simulink model "MCLV2_dsPIC33EP256MC506_externalOpAmp_DataLog_R2017a"  (Simulink 8.9)
settings: Solver=FixedStepDiscrete  StartTime=0.0  StopTime=inf  FixedStep=.00005  RelTol=1e-3  EnableMultiTasking=on
undefined symbols (not defined in the file): A4, A8, B5, B6, C10, C5, C6, D5, DiscIntNeverNeededParam, F0, F1, Max, ms, P20, P24, P53, P54, P97, Pin, PWMmax, Resol, us
libraries: MCHP_Blockset x19, simulink x16, simulink_need_slupdate x1
(part 1 of 2)
Description:
  | MCLV V2 board connected to DC motor through PWM [1 2]
  | PIM 33EP256MC506 with internal Op-Amp (populated with resistances)
  | 
  | LED D2 blink at 5Hz. LED D1 is the CPU busy flag
settings Model: SuppressorTable="22 serialization::archive 15 0 6 0 0 3 8 0 0 0 0 6 0 0 1 0 94 MCLV2_dsPIC33EP256MC506_externalOpAmp_DataLog_R2017a/Steps Large1/Counter Limited 0-1 @ 1.25Hz 0 6 0 0 2 8 0 0 0 0 6 40 SimulinkFixedPoint:util:Overflowoccurred 0 0 0 6 0  0  0 0 0 0 8 20160608 0 0 0 15 23 17 0 1 41 Simulink:DataType:WarningOverFlowDetected 0 0 0  0  8 20160608 0 15 23 17 0 1 1 0 73 MCLV2_dsPIC33EP256MC506_externalOpAmp_DataLog_R2017a/Counter Free-Running 2 8 0 40 SimulinkFixedPoint:util:Overflowoccurred 0 0 0  0  8 20160523 0 10 57 55 0 1 41 Simulink:DataType:WarningOverFlowDetected 0 0 0  0  8 20160523 0 10 57 55 0 1 1 0 93 MCLV2_dsPIC33EP256MC506_externalOpAmp_DataLog_R2017a/Steps Large/Counter Limited 0-1 @ 1.25Hz 2 8 0 40 SimulinkFixedPoint:util:Overflowoccurred 0 0 0  0  8 20160608 0 15 23 17 0 1 41 Simulink:DataType:WarningOverFlowDetected 0 0 0  0  8 20160608 0 15 23 17 0 1"  Creator=R.Delpoux & L.Kerhuel  LastModifiedBy=Lubin Kerhuel
settings DataIOCC: LimitDataPoints=off  SaveFormat=Dataset  SignalLoggingSaveFormat=Dataset
settings OptimizationCC: DefaultParameterBehavior=Inlined  DefaultUnderspecifiedDataType=single  BooleansAsBitfields=on  PassReuseOutputArgsAs=Individual arguments  LifeSpan=auto
settings DebuggingCC: UnderspecifiedInitializationDetection=Simplified  MergeDetectMultiDrivingBlocksExec=error  MultiTaskCondExecSysMsg=none  ParameterOverflowMsg=warning  ParameterTunabilityLossMsg=error  FcnCallInpInsideContextMsg=error  StateNameClashWarn=none  SFUnexpectedBacktrackingDiag=error  SFNoUnconditionalDefaultTransitionDiag=error  SFExecutionAtInitializationDiag=warning
settings HardwareCC: ProdBitPerInt=16  ProdBitPerPointer=16  ProdBitPerSizeT=16  ProdBitPerPtrDiffT=16  ProdLargestAtomicInteger=Integer  ProdIntDivRoundTo=Zero  ProdEndianess=LittleEndian  ProdWordSize=16  ProdHWDeviceType=Generic->Custom
settings ModelReferenceCC: ModelReferenceNumInstancesAllowed=Single  PropagateSignalLabelsOutOfModel=on
settings SFSimCC: MATLABDynamicMemAlloc=off
settings RTWCC: SystemTargetFile=MCHP_dsPIC_stf.tlc  TemplateMakefile=MCHP_dsPIC.tmf  Description=Microchip Embedded Target PIC24 dsPIC30 dsPIC33 (real-time)  GenerateReport=on  IncludeHyperlinkInReport=on  LaunchReport=on  GenerateTraceInfo=on  GenerateTraceReport=on  GenerateTraceReportSl=on  GenerateTraceReportSf=on  GenerateTraceReportEml=on  GenerateCodeReplacementReport=on
settings CodeAppCC: ForceParamTrailComments=on  IgnoreCustomStorageClasses=off  MaxIdLength=255  OperatorAnnotations=on  SimulinkDataObjDesc=on  SFDataObjDesc=on  MATLABFcnDesc=on  InsertBlockDesc=on  MATLABSourceComments=on
settings STFCustomTargetCC: TargetLibSuffix=_lib.a  CodeReplacementLibrary=Microchip Code Replacement Library for dsPIC  MultiwordLength=256  IncludeMdlTerminateFcn=off  CombineOutputUpdateFcns=on  CombineSignalStateStructs=on  SuppressErrorStatus=on  ERTCustomFileBanners=on  SupportContinuousTime=off  RemoveResetFunc=on  MATLABClassNameForMDSCustomization=Simulink.SoftwareTarget.ERTCustomization  GRTInterface=off  SystemTargetFile=MCHP_dsPIC_stf.tlc
settings ERTTargetCC: TargetLibSuffix=_lib.a  CodeReplacementLibrary=Microchip Code Replacement Library for dsPIC  ParMdlRefBuildCompliant=off  CompOptLevelCompliant=off  ConcurrentExecutionCompliant=off  IncludeMdlTerminateFcn=off  CombineSignalStateStructs=on  SuppressErrorStatus=on  SupportNonInlinedSFcns=on  ModelStepFunctionPrototypeControlCompliant=off  CPPClassGenCompliant=off  UseToolchainInfoCompliant=off  ExtModeStaticAllocSize=500  InlinedParameterPlacement=NonHierarchical  ERTSrcFileBannerTemplate=MCHP_dsPIC_code_template.cgt  ERTHdrFileBannerTemplate=MCHP_dsPIC_code_template.cgt  ERTDataSrcFileTemplate=MCHP_dsPIC_code_template.cgt  ERTDataHdrFileTemplate=MCHP_dsPIC_code_template.cgt  ERTCustomFileTemplate=MCHP_main.tlc
settings CustomProperty: DataType=string  Value=33EP256MC506
settings EnumStrPairs: String=elf
settings ConfigComp: CovMetricSettings=dwe  CovHtmlReporting=off  CovSaveCumulativeToWorkspaceVar=off  CovSaveSingleToWorkspaceVar=off  CovExternalEMLEnable=on

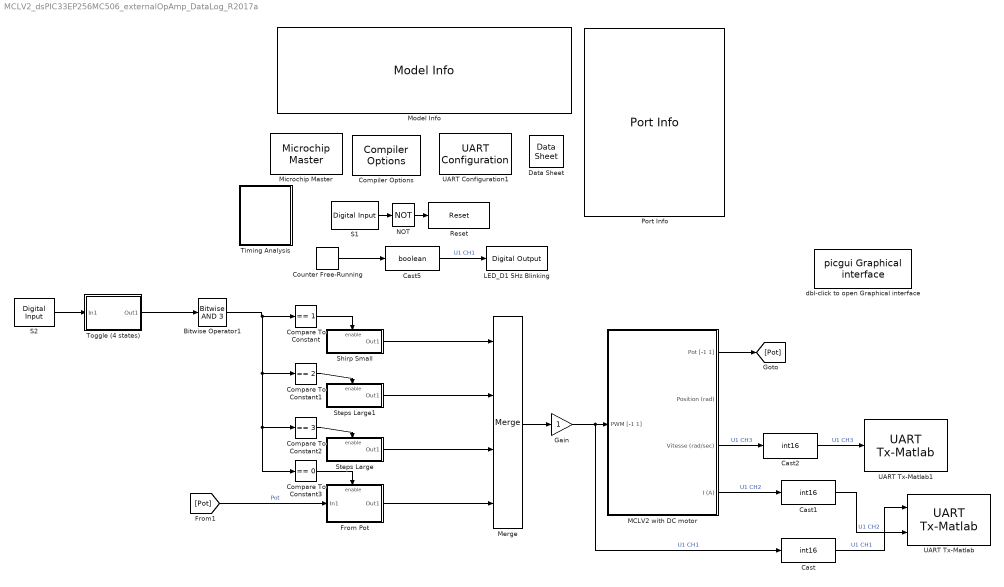
== system MCLV2_dsPIC33EP256MC506_externalOpAmp_DataLog_R2017a ==
  Bitwise Operator1 : simulink/Logic and Bit Operations/Bitwise Operator  logicop=AND  UseBitMask=on  BitMask=3  BitMaskRealWorld=Stored Integer
  Cast : DataTypeConversion  OutDataTypeStr=int16  ConvertRealWorld=Stored Integer (SI)
  Cast1 : DataTypeConversion  OutDataTypeStr=int16  ConvertRealWorld=Stored Integer (SI)
  Cast2 : DataTypeConversion  OutDataTypeStr=int16  ConvertRealWorld=Stored Integer (SI)
  Cast5 : DataTypeConversion  OutDataTypeStr=boolean
  Compare To Constant : simulink/Logic and Bit Operations/Compare To Constant  relop===  const=1  OutDataTypeStr=boolean
  Compare To Constant1 : simulink/Logic and Bit Operations/Compare To Constant  relop===  const=2  OutDataTypeStr=boolean
  Compare To Constant2 : simulink/Logic and Bit Operations/Compare To Constant  relop===  const=3  OutDataTypeStr=boolean
  Compare To Constant3 : simulink/Logic and Bit Operations/Compare To Constant  relop===  const=0  OutDataTypeStr=boolean
  Compiler Options : MCHP_Blockset/System Configuration/Compiler Options  Priority=1  LATEST_CMPLR=on  COMP_LIST=Dynamic Options  COMP_LIST_TXT=xc16 - v1.35  USE_64BIT_DOUBLE=off  MCHP_MULTITHREAD_COMPILATION=on  UseCustom_LinkerScript=off  MCHP_MASTERLINK=MCLV2_dsPIC33EP256MC506_externalOpAmp_DataLog_R2017a/Microchip Master  OPTIMIZATION_LEVEL=1  MPLAB_LINKLIB=default  MPLAB_LINKLIB1=default  UNROLL_LOOPS=on  OMIT_FRAME_POINTER=off  PROCEDURAL_ABSTRACTION=off  MCONST=in code memory  MDATA=Use only memory below address 8192 (faster)  MSCALAR=Use only memory below address 8192 (faster)  MCODE=is less than 32768 (faster)  HEAP_SIZE=0  OMF=elf  DEBUG_INFO=on  AssemblyListing=on  ProduceHexOutput=off
      settings: SourceProductName=MPLAB Device Blocks for Simulink
  Counter Free-Running : simulink/Sources/Counter Free-Running  NumBits=1  tsamp=.1
  Data Sheet : MCHP_Blockset/System Info/Data Sheet  DOC_Type=datasheet  DOC_MCHP_Id=33FJ64MC802  DOC_FileLastCheckTime=[0 0 0 0 0 0]  cpy_MCHP_Id=33EP256MC506  MCHP_MASTERLINK=MCLV2_dsPIC33EP256MC506_externalOpAmp_DataLog_R2017a/Microchip Master
      settings: AttributesFormatString=%<cpy_MCHP_Id>  SourceProductName=MPLAB Device Blocks for Simulink
  From Pot : Subsystem
  Gain : Gain  SaturateOnIntegerOverflow=on  OutDataTypeStr=Inherit: Same as input
  LED_D1 5Hz Blinking : MCHP_Blockset/Digital IO/Digital Output  PORT=Dynamic Options  PORT_TXT="D   [ 5  6  8 ]"  PIN=6  PACK=off  SIMULTANEOUS=off  READPREVIOUS=off  ORDERING=None  SampleTime=-1  MCHP_MASTERLINK=MCLV2_dsPIC33EP256MC506_externalOpAmp_DataLog_R2017a/Microchip Master
      settings: SourceProductName=MPLAB Device Blocks for Simulink
  MCLV2 with DC motor : Subsystem
  Merge : Merge  Inputs=4
  Microchip Master : MCHP_Blockset/System Configuration/Microchip Master  Priority=1  PICREF=33EP256MC506  TIMESTEP_REF=ADC  BUSYFLAG=Dynamic Options  BUSYFLAG_TXT=None  PWRTEN=Not used  BOREN=Disable  BODENV=2.7V  BORV=Not used  FPWRT=128ms  DSBOREN=Enable ZPBOR during Deep Sleep Mode  DSLPBOR=Not used  MCLRE=Enabled  SMCLR=MCLR pin generates a normal system Reset  PMDL1WAY=Allow only one reconfiguration  RSTPRI=Device will obtain reset instruction from Primary flash  TEMP=Not used  SOSCSRC=Not used  SOSCSEL=Not used  IOL1WAY=Allow only one reconfiguration  ALTVREF=Not used  DISUVREG=Not used  DSSWEN=Not used  LPCFG=Not used  RTCBAT=Not used  VBTBOR=Not used  WUTSEL=Not used  POWERSAVE=off  FNOSC=Primary Oscillator (XT; HS; EC)  FPR=ECIO w/ PLL 16x  FOSFPR=HS3 w/PLL 16x  FOS=Primary Oscillator  FRANGE=High Range  OSCILLATOR_SELECT=Crystal / Ceramic resonator  OSCILLATOR_SELECT_spd=Crystal / Ceramic resonator  QUARTZ=8e6  QUARTZ_spd=8e6  POSCGAIN=2x gain setting  POSCBOOST=Boost the kick start of the oscillator  SOSCGAIN=2x gain setting  SOSCBOOST=Boost the kick start of the oscillator  ACTIV_PLL=on  ACTIV_PLL_spd=on  MIPS_DESIRED=70e6  MIPS_DESIRED_spd=70e6  FPLLMUL=Not used  FPLLIDIV=8x Divider  POSCFREQ=Not used  POSCMD=XT Crystal Oscillator Mode  POSCMOD=Primary osc disabled  MIPS=70 * 1e6  ACLKCON=Optimized for PWM resolution & ADC conversion speed  FPLLODIV=32x Divider  PLLKEN=Clock switch to PLL source will wait until the PLL lock signal is valid.  FCKSM=Clock switching is enabled;Fail-safe Clock Monitor is disabled  FCKSMEN=Sw Disabled; Mon Disabled  IESO=Start up with FRC; then switch  DSWDTPS=1:2^36  FWDTEN=Disable  FWDTWINSZ=Window size is 25%  FWPSA=1:512  FWPSA0=1:128  FWPSB=1:16  WDT=Disable  WDTPOST=1:32768  WDTPRE=1:128  WDTPS=1:1048576  WINDIS=Watchdog Timer in Non-Window mode  WWDTEN=Non-Window mode  DSWDTEN=Enable DSWDT during Deep Sleep Mode  DSWDTOSC=Select LPRC as DSWDT Reference clock  FPBDIV=Not used  FSOSCEN=Enable SOSC  LPRCSEL=Not used  OSCIOFCN=Not used  OSCIOFNC=general purpose digital I/O pin  LVRCFG=Not used  PLL_96MHZ=Not used  PLL96MHZ=Not used  PLLDIV=Not used  WDTCLK=Not used  WDTCMX=Not used  WDTWIN=WDT Window is 25% of WDT period  APL=Aux Flash Code protect is disabled  APLK=Aux Flash Write Protection or Code Protection is Enabled  AWRP=Auxiliary program memory is not write-protected  BSS=No Boot program Flash segment  BWP=Not used  BWRP=Boot Segment may be written  CP=Protection Disabled  EBS=No Boot EEPROM  ESS=No Segment Data EEPROM  GCP=General Segment Code protect is Disabled  GSS=General Segment Code protect is Disabled  GSS0=Not used  GSSK=General Segment Write Protection or Code Protection is Enabled  GWRP=General Segment may be written  PWP=Not used  RBS=No Boot RAM  RSS=No Secure RAM  SSS=No Secure Segment  SWRP=Secure segment may be written  WPCFG=Not used  WPDIS=Not used  WPEND=Not used  WPFP=Not used  ICESEL=Communicate on PGEC1/PGED1  ICS=Communicate on PGEC2 and PGED2  JTAGEN=Disable  COE=Not used  RES=Not used  DEBUG=Debugger is disabled  BACKBUG=Not used  BKBUG=Not used  ALTI2C=I2C mapped to SDA1/SCL1 pins  ALTI2C1=I2C1 mapped to SDA1/SCL1 pins  ALTI2C2=I2C2 mapped to SDA2/SCL2 pins  ALTQIO=QEA1; QEB1; INDX1 are selected as inputs to QEI1  ALTSS1=SS1A is selected as the I/O pin for SPI1  CMPPOL0=Hysteresis is applied to falling edge  CMPPOL1=Hysteresis is applied to falling edge  FCANIO=Not used  FETHIO=Default Ethernet I/O  FMIIEN=MII Enabled  FSRSSEL=Not used  FUSBIDIO=Controlled by the USB Module  FVBUSONIO=Not used  HPOL=PWM module high side output pins have active-high output polarity  HYST0=45 mV Hysteresis  HYST1=45 mV Hysteresis  I2C1SEL=Not used  LPOL=PWM module low side output pins have active-high output polarity  PWMPIN=PWM module pins controlled by PORT register at device Reset  RTCOSC=Not used  UPLLEN=USB PLL Disabled  UPLLIDIV=Not used  ATMOD8=Not used  ALTPMP=Not used  I2C2SEL=Not used  ALTADREF=Not used  ALTCVREF=Not used  PWMLOCK=PWM registers may be written without key sequence  MCHP_TIMER_RESULT=[ ]  MCHP_PLLRegisters="[5    243  16385     -1]"  MCHPVAR=MCHP.fcy.MIPS=70000000;MCHP.fcy.SYSCLK=70000000;MCHP.fcy.ADC=70000000;MCHP.fcy.Comparator=70000000;MCHP.fcy.I2C=70000000;MCHP.fcy.SPI=70000000;MCHP.fcy.UART=70000000;MCHP.fcy.Timers=70000000;MCHP.fcy.OC=70000000;MCHP.fcy.IC=70000000;MCHP.fcy.Ports=70000000;MCHP.fcy.QEI=70000000;MCHP.PowerSave=0;MCHP.TimeStepFactor=-20000;MCHP.TimeStep_Timer=-1;MCHP.NTIMERS=5;MCHP.id.name='33EP256MC506';MCHP.id.N=reshape([33 256 506],1,3);MCHP.id.L=reshape({ 'EP','MC',''},1,3);MCHP.id.Arch=3;MCHP.periph.PPS.reg_RPINRx=reshape([-1 1 1 -1 -1 -1 1 -1 -1 -1 -1 -1 -1 -1 1 1 1 1 -1 -1 -1 -1 -1 -1 1 1 -1 -1 1 1 1 1 -1 -1 -1 -1 1 -1 1 -1 -1 -1 -1 -1 1 1 1 -1 -1 -1 -1 -1 1 -1 -1 -1 -1 -1 -1 -1 -1 -1 -1 -1 -1 -1 -1 -1 -1 -1 -1 -1 -1 -1 -1 1 -1 1 1 1],1,80);MCHP.PPS.dsPIC.RP=reshape([-1 -1 -1 -1 -1 -1 -1 -1 -1 -1 -1 -1 -1 -1 -1 -1 -1 -1 -1 -1 4 -1 -1 -1 -1 -1 -1 -1 -1 -1 -1 -1 -1 -1 -1 19 20 21 22 23 24 25 26 27 -1 -1 -1 -1 -1 -1 -1 -1 -1 -1 38 39 40 41 -1 -1 -1 -1 -1 -1 -1 -1 -1 -1 -1 -1 -1 -1 -1 -1 -1 -1 -1 -1 -1 -1 -1 -1 -1 -1 -1 -1 -1 -1 -1 -1 -1 -1 -1 -1 -1 -1 -1 81 -1 -1 -1 -1 -1 -1 -1 -1 -1 -1 -1 -1 -1 -1 -1 -1 -1 -1 -1 -1 102 -1 104],1,121);MCHP.PPS.dsPIC.RPI=reshape([-1 -1 -1 -1 -1 -1 -1 -1 -1 -1 -1 -1 -1 -1 -1 -1 -1 -1 -1 -1 -1 -1 -1 -1 8 9 -1 11 12 -1 -1 -1 16 17 18 -1 -1 -1 -1 -1 -1 -1 -1 -1 28 29 30 31 -1 -1 -1 35 36 37 -1 -1 -1 -1 42 -1 -1 -1 -1 -1 -1 -1 -1 -1 -1 -1 -1 -1 -1 -1 -1 -1 -1 -1 -1 -1 -1 -1 -1 -1 -1 -1 -1 -1 -1 -1 -1 -1 -1 -1 78 79 80 -1 -1 -1 -1 -1 -1 -1 -1 -1 -1 -1 -1 -1 -1 -1 -1 -1 -1 -1 -1 -1 -1 103 -1 105],1,122);MCHP.PPS.dsPIC.RPINR_list=reshape({ '1','INT1','INT2','INT3','INT4','T1CK','T2CK','T3CK','T4CK','T5CK','T6CK','T7CK','T8CK','T9CK','IC1','IC2','IC3','IC4','IC5','IC6','IC7','IC8','OCFA','OCFB','FLT1','FLT2','FLT3','FLT4','QEA1','QEB1','INDX1','HOME1','QEA2','QEB2','INDX2','HOME2','U1RX','U1CTS','U2RX','U2CTS','SDI1','SCK1_in','SS1_in','44','SDI2','SCK2_in','SS2_in','48','CSDIR','CSCK','COFS','52','C1RX','C2RX','U3RX','U3CTS','U4RX','U4CTS','SDI3','SCK3_in','SS3_in','62','SDI4','SCK4_in','SS4_in','66','IC9','IC10','IC11','IC12','IC13','IC14','IC15','IC16','OCFC','SYNCI1','SYNCI2','DTCMP1','DTCMP2','DTCMP3','DTCMP4','DTCMP5','DTCMP6','DTCMP7','FLT5','FLT6','FLT7','FLT8','89','SENT1','SENT2','92'},1,92);MCHP.PPS.dsPIC.RPOR_list=reshape({ '1','U1TX','U1RTS','U2TX','U2RTS','SDO1','SCK1_out','SS1_out','SDO2','SCK2_out','SS2_out','CSDO','CSCK','COFS','C1TX','C2TX','OC1','OC2','OC3','OC4','OC5','OC6','OC7','OC8','C1OUT','C2OUT','C3OUT','U3TX','U3RTS','U4TX','U4RTS','SDO3','SCK3_out','SS3_out','SDO4','SCK4_out','SS4_out','OC9','OC10','OC11','OC12','OC13','OC14','OC15','OC16','SYNCO1','SYNCO2','QEI1CCMP','QEI2CCMP','REFCLK','C4OUT','C5OUT','52','53','54','55','56','SENT1','SENT2'},1,59);MCHP.PPS.map_RPnR_RPORx=reshape([20 35 36 37 38 39 40 41 42 43 54 55 56 57 -1 97 -1 118 120],1,19);MCHP.Rx=reshape([13 15 21 -1 -1 58 -1 -1 -1 -1 -1 14 16 22 -1 -1 59 -1 -1 -1 -1 -1 -1 17 23 -1 -1 -1 -1 -1 -1 -1 -1 -1 18 35 -1 -1 -1 -1 -1 -1 -1 -1 33 32 36 -1 -1 -1 -1 -1 -1 -1 -1 -1 43 37 53 -1 -1 -1 -1 -1 -1 -1 -1 44 50 54 -1 -1 4 -1 -1 -1 -1 1 46 51 -1 -1 -1 5 -1 -1 -1 -1 31 48 52 42 -1 -1 6 -1 -1 -1 -1 34 49 55 -1 -1 -1 8 -1 -1 -1 -1 64 60 45 -1 -1 -1 -1 -1 -1 -1 -1 12 61 24 -1 -1 -1 -1 -1 -1 -1 -1 11 62 39 -1 27 -1 -1 -1 -1 -1 -1 -1 63 47 -1 28 -1 -1 -1 -1 -1 -1 -1 2 -1 -1 29 -1 -1 -1 -1 -1 -1 -1 3 40 -1 30 -1 -1 -1 -1 -1 -1],11,16);MCHP.ADC.ANtype=reshape([3 0],1,2);MCHP.ADC.ADCONx=reshape([47103 59391 40959 263 0 0],1,6);MCHP.ADC.ADCHS_0=reshape([40863 1799],1,2);MCHP.ADC.Flags=reshape([1 0],1,2);MCHP.ADC.Buffer=reshape([16 -1],1,2);MCHP.ADC.port=reshape([0 1 16 17 18 19 32 33 34 11 12 43 76 77 78 79 -1 -1 -1 -1 -1 -1 -1 -1 -1 -1 -1 -1 -1 -1 -1 -1 -1 -1 -1 -1 -1 -1 -1 -1 -1 -1 -1 -1 -1 -1 -1 -1 -1 -1 -1 -1 -1 -1 -1 -1 -1],1,57);MCHP.ADC.port_ALT=reshape([-1 -1 -1 -1],1,4);MCHP.ADC.port_VrefP=17;MCHP.ADC.port_VrefM=16;MCHP.ADC.port_AVdd=-1;MCHP.ADC.port_AVss=-1;MCHP.ADC.ADCDATA=reshape([0 0 0 0 0 0 0 0 0 0 0 0 0 0 0 0 0 0 0 0 0 0 0 0 0 0 0 0 0 0 0 0 0 0 0 0 0 0 0 0 0 0 0 0 0 0 0 0 0 0 0 0 0 0 0 0 0],1,57);MCHP.memory.RAM=32768;MCHP.memory.RAM_XBegin=4096;MCHP.memory.RAM_YBegin=20480;MCHP.memory.RAM_dma=reshape([-1 -1],1,2);MCHP.memory.FLASH_ECC=0;MCHP.DMA.Num=4;MCHP.DMA.CNTmax=16383;MCHP.QEI.QEICONx=reshape([49023 -1 -1 -1 -1 -1],1,6);MCHP.QEI.QEItype=1;MCHP.QEI.Port_QEI_INDX=reshape([-1 -1],1,2);MCHP.QEI.Port_QEI_QEA=reshape([-1 -1],1,2);MCHP.QEI.Port_QEI_QEB=reshape([-1 -1],1,2);MCHP.QEI.Port_QEI_UPDN=reshape([-1 -1],1,2);MCHP.INT.Port=reshape([23 32767 32767 -1 -1],1,5);MCHP.PWM_HS.Flags=reshape([3 1 0],1,3);MCHP.PWM.port_FLT=reshape([-1 -1 -1 34 43 -1 -1 -1 -1 -1 -1 -1 -1 -1 -1 -1 -1 -1 -1 -1 -1 -1 -1 -1 -1 -1 -1 -1 -1 -1 -1 -1 20],1,33);MCHP.PWM.PWMRef=-1;MCHP.PWM.Flag=0;MCHP.PWM.Port_PWM_l=reshape([31 -1 29 -1 27 -1 -1 -1 -1 -1 -1 -1 -1 -1 -1 -1 -1 -1 -1 -1 -1 -1 -1 -1],2,12);MCHP.PWM.Port_PWM_h=reshape([30 -1 28 -1 26 -1 -1 -1 -1 -1 -1 -1 -1 -1 -1 -1 -1 -1 -1 -1 -1 -1 -1 -1],2,12);MCHP.IC.Port=reshape([32767 32767 32767 32767 0 0 0 0 0 0 0 0 0 0 0 0],1,16);MCHP.IC.type=1;MCHP.OC.Port=reshape([32767 32767 32767 32767 0 0 0 0 0 0 0 0 0 0 0 0],1,16);MCHP.OC.type=1;MCHP.CN.Port=reshape([-1 -1 -1 -1 -1 -1 -1 -1 -1 -1 -1 -1 -1 -1 -1 -1 -1 -1 -1 -1 -1 -1 -1 -1 -1 -1 -1 -1 -1 -1 -1 -1 -1 -1 -1 -1 -1 -1 -1 -1 -1 -1 -1 -1 -1 -1 -1 -1 -1 -1 -1 -1 -1 -1 -1 -1 -1 -1 -1 -1 -1 -1 -1 -1 -1 -1 -1 -1 -1 -1 -1 -1 -1 -1 -1 -1 -1 -1 -1 -1 -1 -1 -1 -1 -1],1,85);MCHP.CN.PullUp=reshape([8083 65535 49151 352 61440 3 960 0 0 0 0],1,11);MCHP.CN.type=1;MCHP.CN.Flag_PullDown=1;MCHP.SPI.Refs=reshape([1 2 0 0 0 0],1,6);MCHP.SPI.SPIxCON1=8191;MCHP.SPI.SPIxCON2=57347;MCHP.SPI.Port_SDI=reshape([9 -1 -1 -1 -1 -1],1,6);MCHP.SPI.Port_SDO=reshape([4 -1 -1 -1 -1 -1],1,6);MCHP.SPI.Port_SCK=reshape([35 -1 -1 -1 -1 -1],1,6);MCHP.SPI.Port_SS=reshape([16 -1 -1 -1 -1 -1],1,6);MCHP.I2C.Refs=reshape([1 2 0 0 0],1,5);MCHP.I2C.I2CxCON=49151;MCHP.I2C.NewRegName=1;MCHP.I2C.Port_SDA=reshape([36 8 -1 -1 -1],1,5);MCHP.I2C.Port_SCL=reshape([37 20 -1 -1 -1],1,5);MCHP.I2C.Port_ASDA=reshape([25 21 -1 -1 -1],1,5);MCHP.I2C.Port_ASCL=reshape([24 22 -1 -1 -1],1,5);MCHP.I2C.Fuse_Port_SCL_SDA=reshape([3 1 4 1 -1 -1 -1 -1 -1 -1],2,5);MCHP.I2C.Fuse_Port_ASCL_ASDA=reshape([3 2 4 2 -1 -1 -1 -1 -1 -1],2,5);MCHP.PGA.Port_PGA1P=reshape([-1 -1 -1 -1],1,4);MCHP.PGA.Port_PGA1N=reshape([-1 -1 -1 -1],1,4);MCHP.PGA.Port_PGA2P=reshape([-1 -1 -1 -1],1,4);MCHP.PGA.Port_PGA2N=reshape([-1 -1 -1 -1],1,4);MCHP.PGA.Num=0;MCHP.HS_AnalogComparator.Port_CMP1=reshape([-1 -1 -1 -1],1,4);MCHP.HS_AnalogComparator.Port_CMP2=reshape([-1 -1 -1 -1],1,4);MCHP.HS_AnalogComparator.Port_CMP3=reshape([-1 -1 -1 -1],1,4);MCHP.HS_AnalogComparator.Port_CMP4=reshape([-1 -1 -1 -1],1,4);MCHP.HS_AnalogComparator.PORT_EXTREFx=reshape([-1 -1],1,2);MCHP.HS_AnalogComparator.Port_DACOUTx=reshape([-1 -1],1,2);MCHP.HS_AnalogComparator.Num=0;MCHP.Comp.Port_CVrefin=-1;MCHP.Comp.Port_CVref=-1;MCHP.Comp.Port_CVref1O=24;MCHP.Comp.Port_CVref2O=4;MCHP.Comp.Port_CxOUT=reshape([32767 32767 32767 32767 -1],1,5);MCHP.Comp.Port_OAxOUT=reshape([17 0 32 -1 -1],1,5);MCHP.Comp.Port_CxINP=reshape([18 1 34 32 -1],1,5);MCHP.Comp.Port_CxINM=reshape([19 43 -1 -1 16 76 -1 -1 33 77 -1 -1 33 -1 -1 -1 -1 -1 -1 -1],4,5);MCHP.Comp.nComp=reshape([4 0 0],1,3);MCHP.Comp.OpAmp=7;MCHP.Comp.CVRCON=reshape([17663 0],1,2);MCHP.CDAC.Port_DACx=reshape([-1 -1 -1],1,3);MCHP.CDAC.nCDAC=0;MCHP.UART.port_Rx=reshape([32767 32767 -1 -1 -1 -1],1,6);MCHP.UART.port_Tx=reshape([32767 32767 -1 -1 -1 -1],1,6);MCHP.UART.port_ARx=reshape([-1 -1],1,2);MCHP.UART.port_ATx=reshape([-1 -1],1,2);MCHP.UART.port_RTS=reshape([34 76 -1 -1 -1 -1],1,6);MCHP.UART.port_CTS=reshape([43 77 -1 -1 -1 -1],1,6);MCHP.UART.reg_UxMODE=reshape([48127 48127 -1 -1 -1 -1],1,6);MCHP.UART.reg_UxSTA=reshape([61439 61439 -1 -1 -1 -1],1,6);MCHP.modsrc.DOS_00794=1;MCHP.modsrc.DOS_00931=1;MCHP.modsrc.DOS_00932=1;MCHP.modsrc.DOS_00942=1;MCHP.modsrc.DOS_00938=1;MCHP.modsrc.DOS_00996=1;MCHP.modsrc.DOS_00997=1;MCHP.modsrc.DOS_00998=1;MCHP.modsrc.DOS_00209=0;MCHP.modsrc.DOS_01555_adc=0;MCHP.modsrc.DOS_01293=1;MCHP.modsrc.DOS_00828=0;MCHP.modsrc.DOS_01116=1;MCHP.modsrc.DOS_01017_RPORx=1;MCHP.modsrc.DOS_01017_RPINRx=1;MCHP.modsrc.DOS_01555_nvm_tsmc18_v2_16bit=0;MCHP.modsrc.DOS_00804=1;MCHP.modsrc.DOS_00826=1;MCHP.modsrc.DOS_01555_TLAK_PMDx=0;MCHP.modsrc.DOS_01555_TLAK_INT_=0;MCHP.modsrc.DOS_00933=1;MCHP.modsrc.DOS_01555=0;MCHP.modsrc.DOS_01555_ptg=0;MCHP.modsrc.DOS_00929=1;MCHP.modsrc.DOS_00958=1;MCHP.modsrc.DOS_01117_PORTx=1;MCHP.modsrc.DOS_00999=0;MCHP.modsrc.DOS_01198=1;MCHP.modsrc.DOS_01041=1;MCHP.modsrc.DOS_00892=1;MCHP.modsrc.DOS_01287_TLAC_PMDx=1;MCHP.modsrc.DOS_01287_TLAC_INT_=1;MCHP.modsrc.DOS_01424=1;MCHP.modsrc.DOS_01332=1;MCHP.modsrc.DOS_01441_i2c_upb_v1_16bit_TLAH=0;MCHP.modsrc.DOS_01482=0;MCHP.modsrc.DOS_02508c11=0;MCHP.modsrc.DOS_01468_PMBA_current_source=0;MCHP.modsrc.DOS_02291_PGA=0;MCHP.modsrc.DOS_01467_Comparator=0;MCHP.modsrc.DOS_01498_TLAY=0;MCHP.modsrc.DOS_02316_nvm_ctrl_v1_16bit=0;MCHP.modsrc.DOS_00993_PLL_120MHz=0;MCHP.modsrc.DOS_01577_cla_clc_upb_v1=0;MCHP.modsrc.DOS_01332_ptg_pc_v1=0;MCHP.modsrc.DOS_00958_pwm_TLAY=0;MCHP.modsrc.TLAY_IOPorts=0;MCHP.modsrc.DOS_00929q=0;MCHP.modsrc.DOS_02415_spi_v5=0;MCHP.modsrc.DOS_RPINRx_16bit_2=0;MCHP.modsrc.DOS_01497_TLAH_PMDx=0;MCHP.modsrc.DOS_02550_TLAL_INT=0;MCHP.modsrc.DOS_00958_pwm_TLAH=0;MCHP.modsrc.DOS_01287_TLAH_INT_=0;MCHP.modsrc.DOS_01113=0;MCHP.modsrc.DOS_01017_PMDx=0;MCHP.modsrc.DOS_00927=0;MCHP.modsrc.DOS_01080=0;MCHP.modsrc.DOS_00794_cpu_16bit_v3=0;MCHP.modsrc.DOS_02359a_sent_j2716_upb_v1=0;MCHP.modsrc.DOS_01520_wdt_dmt_upb_v1_16bit=0;MCHP.modsrc.DOS_02192_TLCD_PMDx=0;MCHP.modsrc.DOS_02192_TLCD_INT_=0;MCHP.modsrc.DOS_02192_cmp=0;MCHP.modsrc.DOS_00958_pwm_TLCD=0;MCHP.modsrc.DOS_02192_PORTx_TLCD=0;MCHP.modsrc.DOS_00936=0;MCHP.modsrc.DOS_00995=0;MCHP.modsrc.DOS_00546=0;MCHP.modsrc.DOS_00474=0;MCHP.modsrc.DOS_02481_WACJ_Config=0;MCHP.modsrc.DOS_02569_pfm_cache_ocp_v1=0;MCHP.modsrc.DOS_02819_pfm_ctrl_32bit_upb_v2=0;MCHP.modsrc.DOS_02674_wdt_upb_v1_32bit=0;MCHP.modsrc.DOS_01520_wdt_dmt_upb_v1=0;MCHP.modsrc.DOS_02869_icd_jtag_bvci_upb_v2=0;MCHP.modsrc.DOS_02823_WACJ_clk_cru_upb_v2=0;MCHP.modsrc.DOS_01423_RPINRx=0;MCHP.modsrc.DOS_02481_RPORx=0;MCHP.modsrc.DOS_02511_pwr_sib_upb_v1_32bit=0;MCHP.modsrc.DOS_02481_WACJ_int_evic_v3=0;MCHP.modsrc.DOS_01500_dma_bvci_v2=0;MCHP.modsrc.DOS_02141_tmr_classa_pb_v2=0;MCHP.modsrc.DOS_02815_tmr_classb_upb_v1=0;MCHP.modsrc.DOS_00740_icap_pb_v1=0;MCHP.modsrc.DOS_00749_ocmp_pb_v1=0;MCHP.modsrc.DOS_01441_i2c_upb_v1_32bit=0;MCHP.modsrc.DOS_01329_spi_pb_v2=0;MCHP.modsrc.DOS_02478_uart_irda_upb_v1_32bit=0;MCHP.modsrc.DOS_02514_dfm_strl_sst_upb_v1=0;MCHP.modsrc.DOS_01427_cmp_control_upb_v1_32bit=0;MCHP.modsrc.DOS_01445_dac_nbit__control_upb_v1_32bit=0;MCHP.modsrc.DOS_01461_afe_ctmu_con_upb_v1=0;MCHP.modsrc.DOS_02472_ppi_pmp16_upb_v1=0;MCHP.modsrc.DOS_02467_gpio_ports_upb_v1=0;MCHP.modsrc.DOS_02508_adc_sar_ctrl_upb_v1_PIC32MK=0;MCHP.modsrc.DOS_02813a_usb_otgcore_pb_v3=0;MCHP.modsrc.DOS_01261_tmr_rtcc_pb_v2=0;MCHP.modsrc.DOS_01475_lpwr_deep_sleep_ctrl_v2=0;MCHP.modsrc.DOS_EIP_00136_ssx_v1=0;MCHP.modsrc.DOS_01152_can_bvci_v1=0;MCHP.modsrc.DOS_02481_WACN_Config=0;MCHP.modsrc.DOS_02823_WACN_clk_cru_upb_v2=0;MCHP.modsrc.DOS_02481_WACN_int_evic_v3=0;MCHP.modsrc.DOS_03554_cmp_control_upb_v2_32bit=0;MCHP.modsrc.DOS_01577_cla_clc_upb_v1_32bit=0;MCHP.modsrc.DOS_03247_can_fd_upb_v2=0;MCHP.modsrc.DOS_02481_WACK_MC_Config=0;MCHP.modsrc.DOS_03247_can_fd_upb_v2_pic32mk=0;MCHP.modsrc.DOS_02481_WACJ_MC_Config=0;MCHP.modsrc.DOS_02481_WACJ_MC_int_evic_v3=0;MCHP.modsrc.DOS_01477_pwm_mc_upb_v1=0;MCHP.modsrc.DOS_01459_ptg_pc_upb_v1_SIC=0;MCHP.modsrc.DOS_01494_qei_32b_upb_v1=0;MCHP.modsrc.DOS_02481_WACN_MC_Config=0;MCHP.modsrc.DOS_02481_WACN_MC_int_evic_v3=0;MCHP.modsrc.DOS_02787_WACD_Config=0;MCHP.modsrc.DOS_00800_dac_4bit_ctrl_pb_v1=0;MCHP.modsrc.DOS_01539_icd_jtag_pb_v2=0;MCHP.modsrc.DOS_02823_clk_cru_upb_v2=0;MCHP.modsrc.DOS_01423_RPORx=0;MCHP.modsrc.DOS_02907_WACD_int_evic_v3=0;MCHP.modsrc.DOS_00734_uart_irda_pb_v1=0;MCHP.modsrc.DOS_00687_tmr_classa_pb_v1=0;MCHP.modsrc.DOS_00745_tmr_classb_pb_v1=0;MCHP.modsrc.DOS_02508_adc_sar_ctrl_upb_v1=0;MCHP.modsrc.DOS_00866_cmp_control_pb_v2=0;MCHP.modsrc.DOS_01114_eth_bvci_v1=0;MCHP.modsrc.DOS_02831_usb_clk_rst_v2=0;MCHP.modsrc.DOS_01643_pfm_cache_ahb_v2=0;MCHP.modsrc.DOS_EIP_00206r5_sqi_v2=0;MCHP.modsrc.DOS_EIP_00124_usb_hs_otgcore_v1=0;MCHP.modsrc.DOS_EIP_00218_math_rng_ahbs_v2=0;MCHP.modsrc.DOS_EIP_00109_ebi_v1=0;MCHP.modsrc.DOS_EIP_00158_crypto_v1=0;MCHP.clock.PBxDIV=-1;  MCHP_CRC=5751430  BTMODE=Not used  RES1=Not used  PLLSS=Not used  RES2=Not used  ALTCMPI=Not used  BOREN1=Not used  ALTRB6=Not used  RETCFG=Not used  DFMCY=Not used  BSS2=No Boot Segment  BSEN=No Boot Segment  CWRP=Configuration Segment may be written  CSS=No Protection (other than CWRP)  AIVTDIS=Disable Alternate Vector Table  BSLIM=Not used  WDTEN=Disable  BTSWP=BOOTSWP instruction is disabled  DBCC=No Cross Connection between DAC outputs  CTXT1=Not Assigned  CTXT2=Not Assigned  SEQNUM=Not used  nSEQNUM=Not used  BOREN0=Enabled  DMTIVT=Not used  DMTCNT=2^8 (256)  DMTEN=Dead Man Timer is Disabled and can be enabled by software  ON=Not used  USERID=Not used  RESERVED1=Not used  PGL1WAY=Allow only one reconfiguration  FPLLRNG=34-68 MHz Input  FPLLICLK=FRC is input to the System PLL  FPLLMULT=PLL Multiply by 128  UPLLFSEL=USB PLL input is 24 MHz  DMTINTV=Window/Interval value is 127/128 counter value  WDTSPGM=WDT stops during Flash programming  FDMTEN=Deadman Timer is disabled  TRCEN=Trace features in the CPU are enabled  BOOTISA=Boot code and Exception code is MIPS32  FECCCON=ECC and Dynamic ECC are disabled (ECCCON bits are writable)  EXTDDRSIZE=Not used  FSLEEP=Flash is powered down when the device is in Sleep mode  DBGPER=Allow CPU access to all permission regions  EJTAGBEN=Normal EJTAG functionality  TSEQ=Not used  CSEQ=Not used
      settings: SourceProductName=MPLAB Device Blocks for Simulink
  Model Info : simulink/Model-Wide Utilities/Model Info  Frame=on  DisplayStringWithTags=|  HorizontalTextAlignment=Center  LeftAlignmentValue=0.5
      | %<ModelName> v%<ModelVersion> - %<Creator>
      | 
      | %<Description>
      | 
      | Lost modified on: %<LastModificationDate>
  NOT : Logic  Operator=NOT  IconShape=distinctive  AllPortsSameDT=off  OutDataTypeStr=boolean
  Port Info : MCHP_Blockset/System Info/Port Info  MCHP_MASTERLINK=MCLV2_dsPIC33EP256MC506_externalOpAmp_DataLog_R2017a/Microchip Master
      settings: SourceProductName=MPLAB® Device Blocks for Simulink®
  Reset : MCHP_Blockset/System Functions/Reset  SampleTime=-1  MCHP_MASTERLINK=UTestBoard_33FJ256GP710A_2/Microchip Master
      settings: SourceProductName=MPLAB Device Blocks for Simulink
  S1 : MCHP_Blockset/Digital IO/Digital Input  PORT=Dynamic Options  PORT_TXT="G   [ 6 : 9 ]"  PIN=6  PACK=off  SIMULTANEOUS=off  ORDERING=None  SampleTime=.1  MCHP_PORT={Digital In}{DIN}2:0:G6;  MCHP_MASTERLINK=MCLV2_dsPIC33EP256MC506_externalOpAmp_DataLog_R2017a/Microchip Master
      settings: SourceProductName=MPLAB Device Blocks for Simulink
  S2 : MCHP_Blockset/Digital IO/Digital Input  PORT=Dynamic Options  PORT_TXT="G   [ 6 : 9 ]"  PIN=7  PACK=off  SIMULTANEOUS=off  ORDERING=None  SampleTime=-1  MCHP_PORT={Digital In}{DIN}2:0:G7;  MCHP_MASTERLINK=MCLV2_dsPIC33EP256MC506_externalOpAmp_DataLog_R2017a/Microchip Master
      settings: SourceProductName=MPLAB Device Blocks for Simulink
  Shirp Small : Subsystem
  Steps Large : Subsystem
  Steps Large1 : Subsystem
  Timing Analysis : Subsystem
  Toggle (4 states) : Subsystem
  UART Configuration1 : MCHP_Blockset/BUS UART/UART Configuration  UART_REF=1  BAUD_Choice=Dynamic Options  BAUD_Choice_TXT="2000000         [-2.78%]"  BAUD_Choice_IR=Dynamic Options  BAUD_Choice_IR_TXT=[]  BAUD_Custom=115200  ALT_IO=on  PIN_RX=Dynamic Options  PIN_RX_TXT=C5 / P53 / Pin[37]  PIN_TX=Dynamic Options  PIN_TX_TXT=F1 / P97 / Pin[59]  MCHP_PORT="{UART1  Rx}{U1RX}3:0:P53;{UART1  Tx}{U1TX}3:1:P97;"  MCHP_MASTERLINK=MCLV2_dsPIC33EP256MC506_externalOpAmp_DataLog_R2017a/Microchip Master  MCHP_COM_ExtPil=off  TX_IMPLEMENTATION=DMA Ping-Pong Mode  TX_IMPLEMENTATION_default=Circular Buffer  TX_INT_PRIORITY=5  TX_INT_WHEN=is empty  TX_INT_WHEN_default=is empty & last char is sent  TX_CIRCULAR_SIZE=128  TX_DMA_CHANNEL="0   (Lowest Priority)"  TX_DMA_SIZE=[3*20]  TX_TASK_PROTECTION=Delay tasks (default)  TX_INTERRUPT_PROTECTION=Do not send on conflict (default)  TX_INTERRUPT_PROTECTION_default=Do not send on conflict (default)  RX_IMPLEMENTATION=Simplest (4 bytes internal buffer only)  RX_IMPLEMENTATION_default=Circular Buffer  RX_INT_PRIORITY=1  RX_INT_WHEN=receive 1 character  RX_CIRCULAR_SIZE=2048  DuplexMode=Full duplex (default)  PIN_RX_Inv=off  PIN_TX_Inv=off  ParityBit=No parity (default)  StopBit=1 stop bit (default)  IRDA=off  FlowControl=None  PIN_CTS=Dynamic Options  PIN_CTS_TXT=A4 / P20 / Pin[33]  PIN_RTS=Dynamic Options  PIN_RTS_TXT=A4 / P20 / Pin[33]  InitSequence_chkbox=off  BAUD_Choice_InitSeq=Dynamic Options  BAUD_Choice_InitSeq_TXT="115200         [-0.06%]"  BAUD_Choice_IR_InitSeq=Dynamic Options  BAUD_Choice_IR_InitSeq_TXT=0  BAUD_Custom_InitSeq=0  InitSequence=['Init done' 10 13]
      settings: SourceProductName=MPLAB® Device Blocks for Simulink®
  UART Tx-Matlab : MCHP_Blockset/BUS UART/UART Tx-Matlab  UART_REF=1  CHANNELS=[1 2 ]  AllOrNothing=on  SampleTime=-1  MCHP_MASTERLINK=MCLV2_dsPIC33EP256MC506_externalOpAmp_DataLog_R2017a/Microchip Master  MCHP_COMPILED_INFO="CompiledSampleTime= [5.0000000000000002396e-05   0 ];CompiledInportDataTypes=[  4   4 ];CompiledInportDataWidth=[1  1];"
      settings: SourceProductName=MPLAB Device Blocks for Simulink
  UART Tx-Matlab1 : MCHP_Blockset/BUS UART/UART Tx-Matlab  UART_REF=1  CHANNELS=[3]  AllOrNothing=on  SampleTime=-1  MCHP_MASTERLINK=MCLV2_dsPIC33EP256MC506_externalOpAmp_DataLog_R2017a/Microchip Master  MCHP_COMPILED_INFO="CompiledSampleTime= [0.0020000000000000000416   0 ];CompiledInportDataTypes=[  4 ];CompiledInportDataWidth=[1];"
      settings: SourceProductName=MPLAB Device Blocks for Simulink
  dbl-click to open Graphical interface : MCHP_Blockset/BUS UART/picgui Graphical interface  Nothing=0
      settings: SourceProductName=MPLAB Device Blocks for Simulink
  wires:
  Gain/1 -> MCLV2 with DC motor/1(PWM [-1 1]), Cast/1  "U1 CH1"
  Counter Free-Running/1 -> Cast5/1
  Cast5/1 -> LED_D1 5Hz Blinking/1  "U1 CH1"
  MCLV2 with DC motor/1(Pot [-1 1]) -> [Pot]
  S2/1 -> Toggle (4 states)/1(In1)
  MCLV2 with DC motor/4(I (A)) -> Cast1/1  "U1 CH2"
  Steps Large1/1(Out1) -> Merge/2
  Bitwise Operator1/1 -> Compare To Constant/1, Compare To Constant1/1, Compare To Constant2/1, Compare To Constant3/1
  Compare To Constant/1 -> Shirp Small/Enable
  Compare To Constant1/1 -> Steps Large1/Enable
  Compare To Constant2/1 -> Steps Large/Enable
  [Pot] -> From Pot/1(In1)  "Pot"
  Compare To Constant3/1 -> From Pot/Enable
  Shirp Small/1(Out1) -> Merge/1
  From Pot/1(Out1) -> Merge/4
  Steps Large/1(Out1) -> Merge/3
  Toggle (4 states)/1(Out1) -> Bitwise Operator1/1
  Merge/1 -> Gain/1
  MCLV2 with DC motor/3(Vitesse (rad/sec)) -> Cast2/1  "U1 CH3"
  Cast1/1 -> UART Tx-Matlab/2  "U1 CH2"
  Cast/1 -> UART Tx-Matlab/1  "U1 CH1"
  NOT/1 -> Reset/1
  S1/1 -> NOT/1
  Cast2/1 -> UART Tx-Matlab1/1  "U1 CH3"

== system MCLV2_dsPIC33EP256MC506_externalOpAmp_DataLog_R2017a/From Pot ==
  In1 : Inport
  Enable : EnablePort
  Gain : Gain  OutDataTypeStr=fixdt(1,16,15)
  Out1 : Outport
  wires:
  In1/1 -> Gain/1
  Gain/1 -> Out1/1  "Duty Cycle"

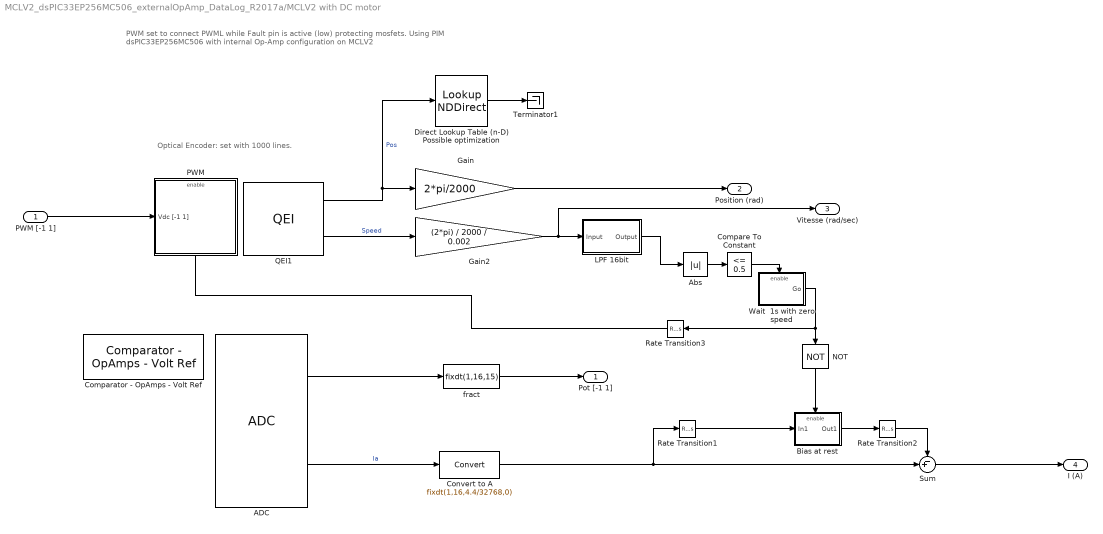
== system MCLV2_dsPIC33EP256MC506_externalOpAmp_DataLog_R2017a/MCLV2 with DC motor ==
  note: PWM set to connect PWML while Fault pin is active (low) protecting mosfets.
      | Using PIM dsPIC33EP256MC506 with internal Op-Amp configuration on MCLV2
  note: Optical Encoder: set with 1000 lines.
  PWM [-1 1] : Inport
  ADC : MCHP_Blockset/Analog IO/ADC  Priority=5  ADC_REF=1  Mode=10 bits (allows exact simultaneous sampling)  FORM="sddd dddd dddd 0000  ==> Signed fractional"  ADC_R="< 5    kOhm"  nSAMPLECHANNELS=CH0 : CH1  nSAMPLECHANNELS_12bits=CH0 only  SIMULTANEOUS=Simultaneously on all Channels  ADxCSS=[13]  MUXA_CH0N=off  MUXA_CH123=Dynamic Options  MUXA_CH123_TXT=OA2 : AN1 : AN2  MUXB_CH0=AN1  MUXB_CH0N=on  MUXB_CH123=Dynamic Options  MUXB_CH123_TXT=OA2 : AN1 : AN2  SequenceRepeat=1  SequenceTiming=are done as fast as possible ; triggered by user define source  SSRC_SSRCG=Dynamic Options  SSRC_SSRCG_TXT=6  Update_BlockOutput=After each trig and conversion sequence  Trig_TimeStep=with each update of the ADC block output  ADC_DMA_CHANNEL=Use Interrupt instead of DMA  SampleTime=5e-05  Info=Total Time for Sample & Conversion : 2.4e-06s including 3.4286e-07s (x 1) sample time.  MCHP_PORT={Analog Input 0}{AN0}15:2:A0;{Analog Input 13}{AN13}15:2:E13;  MCHP_MASTERLINK=MCLV2_dsPIC33EP256MC506_externalOpAmp_DataLog_R2017a/Microchip Master  ADC_TIMING=[2.4000000000000003149e-06]
      settings: SourceProductName=MPLAB Device Blocks for Simulink
  Abs : Abs
  Bias at rest : Subsystem  TreatAsAtomicUnit=on
  Comparator - OpAmps - Volt Ref : MCHP_Blockset/Analog IO/Comparator - OpAmps - Volt Ref  MCHP_params=s.CVR1OE=0;s.CVR2OE=0;s.VREFSEL=0;s.RLaddle=reshape([1 1],1,2);s.AVdd=reshape({ '3.3','3.3'},1,2);s.AVss=reshape({ '0','0'},1,2);s.CVRSS=reshape([0 0],1,2);s.CON_OPMODE_CPOL=reshape([0 3 0 0 0],1,5);s.OutputPort_COE_RP=reshape({ 'B1 / Pin[16] / OA1OUT / AN3 / OA1OUT','A0 / Pin[13] / OA2OUT / AN0 / OA2OUT','C0 / Pin[21] / OA3OUT / AN6 / OA3OUT','None','None'},1,5);s.InputP_CREF=reshape([0 0 0 0 0],1,5);s.InputN_CCH=reshape([0 0 0 0 0],1,5);s.Trigger_EventInterrupt_EVPOL=reshape([0 0 0 0 0],1,5);s.BlockOutputEvent=reshape([0 0 0 0 0],1,5);s.BlockOutputState=reshape([0 0 0 0 0],1,5);s.IntPriority=5;s.FilterFreq=reshape([1e+10 1e+10 1e+10 1e+10 1e+10],1,5);s.Blanking=reshape([1 1 1 1 1],1,5);s.BlankingSignal=reshape({ ' - ',' - ',' - ',' - ',' - ',' - ',' - ',' - ',' - ',' - ',' - ',' - ',' - ',' - ',' - '},3,5);s.BlankingTruthTable=reshape([-1 -1 -1 -1 -1 -1 -1 -1 -1 -1 -1 -1 -1 -1 -1 -1 -1 -1 -1 -1 -1 -1 -1 -1 -1 -1 -1 -1 -1 -1 -1 -1 -1 -1 -1 -1 -1 -1 -1 -1 -1 -1 -1 -1 -1 -1 -1 -1 -1 -1 -1 -1 -1 -1 -1 -1 -1 -1 -1 -1 -1 -1 -1 -1 -1 -1 -1 -1 -1 -1 -1 -1 -1 -1 -1 -1 -1 -1 -1 -1 -1 -1 -1 -1 -1 -1 -1 -1 -1 -1 -1 -1 -1 -1 -1 -1 -1 -1 -1 -1 -1 -1 -1 -1 -1 -1 -1 -1 -1 -1 -1 -1 -1 -1 -1 -1 -1 -1 -1 -1 -1 -1 -1 -1 -1 -1 -1 -1 -1 -1 -1 -1 -1 -1 -1 -1 -1 -1 -1 -1 -1 -1 -1 -1 -1 -1 -1 -1 -1 -1 -1 -1 -1 -1 -1 -1 -1 -1 -1 -1 -1 -1 -1 -1 -1 -1 -1 -1 -1 -1 -1 -1 -1 -1 -1 -1 -1 -1 -1 -1 -1 -1 -1 -1 -1 -1 -1 -1 -1 -1 -1 -1 -1 -1 -1 -1 -1 -1 -1 -1 -1 -1 -1 -1 -1 -1 -1 -1 -1 -1 -1 -1 -1 -1 -1 -1 -1 -1 -1 -1 -1 -1 -1 -1 -1 -1 -1 -1 -1 -1 -1 -1 -1 -1 -1 -1 -1 -1 -1 -1],16 ,3 ,5);  S_INPUT="[5  5]"  S_OUTPUT=[5]  S_INPUT_Size="[2  2]"  S_OUTPUT_Size=[4]  SampleTime=-1  MCHP_MASTERLINK=MCLV2_dsPIC33EP256MC506_externalOpAmp_DataLog_R2017a/Microchip Master  MCHP_PORT={Op-Amp Output 2}{OA2(out)}14:2:A0;{Op-Amp2 V+}{OA2 V+}14:2:A1;{Op-Amp2 V-}{OA2 V-}14:2:B0;  ORDERING=0
      settings: SourceProductName=MPLAB Device Blocks for Simulink
  Compare To Constant : simulink/Logic and Bit Operations/Compare To Constant  relop=<=  const=0.5  OutDataTypeStr=boolean
  Convert to A : DataTypeConversion  OutDataTypeStr=fixdt(1,16,4.4/32768,0)  ConvertRealWorld=Stored Integer (SI)
  Direct Lookup Table (n-D) Possible optimization : LookupNDDirect  NumberOfTableDimensions=1  Table=[0:(1000-1)]*2*pi/1000  TableDataTypeStr=fixdt(1,16,5)
      settings: LockScale=on
  Gain : Gain  Gain=2*pi/2000  OutDataTypeStr=fixdt(1,16,5)
  Gain2 : Gain  Gain=(2*pi) / 2000 / 0.002  OutDataTypeStr=fixdt(1,16,5)  LockScale=on
  "LPF 16bit  " : Subsystem  Tag=FilterWizardSubSystem
      settings: ErrorFcn=dspFilterRealizedInBasicElemsAlgLoopErrFcnCallback
  NOT : Logic  Operator=NOT  IconShape=distinctive  AllPortsSameDT=off  OutDataTypeStr=boolean
  PWM : Subsystem
  QEI1 : MCHP_Blockset/QEI/QEI  QEI_REF=1  QEI_MODE=Quadrature Encoder  QEI_x2mode=off  QEI_PulseCountDir=Down  PIN_QEA=Dynamic Options  PIN_QEA_TXT=A8 / P24 / Pin[31]  PIN_QEB=Dynamic Options  PIN_QEB_TXT=C6 / P54 / Pin[50]  SWPAB=off  QEAPOL=off  QEBPOL=off  SampleTime=.002  INDXxCNT_Output=is not an output  POSxCNT_Output=is a 16 bits unsigned block output  RESET_Input=off  PIMOD_mode=position is cyclique between user defined boundaries  PIMOD_modeB=Never reset position  PIMOD_reset=on next INDEX event  PIN_INDEX=Dynamic Options  PIN_INDEX_TXT=A4 / P20 / Pin[33]  IMV=QEA = 1 and QEB = 0  IMV_x2=QEA = 1  PIN_HOME=Dynamic Options  PIN_HOME_TXT=A4 / P20 / Pin[33]  QEIxLEC_GEC=[0 1999]  QEIxIC=0  PCIIRQ=off  IDXPOL=off  HOMPOL=on  VELxCNT_Output=is a 16 bits signed block output  INTxHLD_Output=is not an output  MaxPeriod=1e-3  FILTREN=on  QFDIV_popup=Dynamic Options  QFDIV_popup_TXT=729.17 kHz  FILTER_CutOffFreq=100e3  PIN_CCMP=Dynamic Options  PIN_CCMP_TXT=A4 / P20 / Pin[33]  MCHP_PORT={QEI1 A}{QEA1}5:0:P24;{QEI1 B}{QEB1}5:0:P54;  MCHP_MASTERLINK=MCLV2_dsPIC33EP256MC506_externalOpAmp_DataLog_R2017a/Microchip Master  QEI_IntPri=5
      settings: SourceProductName=MPLAB Device Blocks for Simulink
  Rate Transition1 : RateTransition  Deterministic=off  OutPortSampleTime=.002
  Rate Transition2 : RateTransition  Deterministic=off
  Rate Transition3 : RateTransition  Deterministic=off
  Sum : Sum  Inputs=-+|  OutDataTypeStr=Inherit: Inherit via back propagation  SaturateOnIntegerOverflow=on  InputSameDT=on
  Terminator1 : Terminator
  Wait  1s with zero speed : Subsystem  TreatAsAtomicUnit=on
  fract : DataTypeConversion  OutDataTypeStr=fixdt(1,16,15)  ConvertRealWorld=Stored Integer (SI)
  Pot [-1 1] : Outport
  Position (rad) : Outport  Port=2
  Vitesse (rad/sec) : Outport  Port=3
  I (A) : Outport  Port=4
  wires:
  Abs/1 -> Compare To Constant/1
  Rate Transition3/1 -> PWM/Enable
  Compare To Constant/1 -> Wait  1s with zero speed/Enable
  Wait  1s with zero speed/1(Go) -> NOT/1, Rate Transition3/1
  PWM [-1 1]/1 -> PWM/1(Vdc [-1 1])
  NOT/1 -> Bias at rest/Enable
  Rate Transition2/1 -> Sum/1
  Rate Transition1/1 -> Bias at rest/1(In1)
  Bias at rest/1(Out1) -> Rate Transition2/1
  Sum/1 -> I (A)/1
  ADC/2 -> Convert to A/1  "Ia"
  Convert to A/1 -> Rate Transition1/1, Sum/2
  "LPF 16bit  "/1(Output) -> Abs/1
  Gain2/1 -> Vitesse (rad/sec)/1, "LPF 16bit  "/1(Input)
  Gain/1 -> Position (rad)/1
  fract/1 -> Pot [-1 1]/1
  QEI1/1 -> Gain/1, Direct Lookup Table (n-D) Possible optimization/1  "Pos"
  ADC/1 -> fract/1
  QEI1/2 -> Gain2/1  "Speed"
  Direct Lookup Table (n-D) Possible optimization/1 -> Terminator1/1

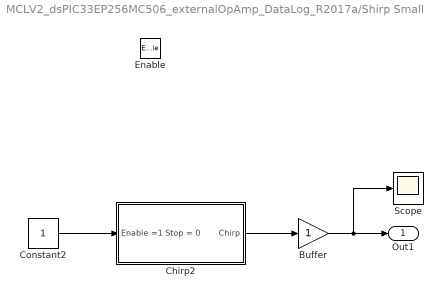
== system MCLV2_dsPIC33EP256MC506_externalOpAmp_DataLog_R2017a/Shirp Small ==
  Enable : EnablePort  StatesWhenEnabling=reset
  Buffer : Gain  OutDataTypeStr=Inherit: Inherit via back propagation  ParamDataTypeStr=Inherit: Same as input
  Chirp2 : Subsystem  mask{Fmax=30, Tend=50, Fs=1000, MaxVal=0.5, MinVal=0.2, StartDelay=2}
      mask prompts: MaxVal "Max value"; MinVal "Min value"
  Constant2 : Constant
  Scope : Scope
  Out1 : Outport
  wires:
  Buffer/1 -> Scope/1, Out1/1
  Chirp2/1(Chirp) -> Buffer/1
  Constant2/1 -> Chirp2/1(Enable =1 Stop = 0)

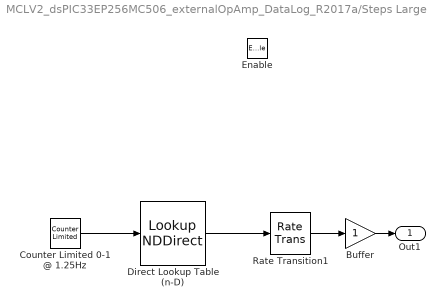
== system MCLV2_dsPIC33EP256MC506_externalOpAmp_DataLog_R2017a/Steps Large ==
  Enable : EnablePort  StatesWhenEnabling=reset
  Buffer : Gain  OutDataTypeStr=Inherit: Same as input  ParamDataTypeStr=Inherit: Same as input
  Counter Limited 0-1 @ 1.25Hz : simulink/Sources/Counter Limited  uplimit=19  tsamp=2.5
  Direct Lookup Table (n-D) : LookupNDDirect  NumberOfTableDimensions=1  Table="round([0 0 10 20 30 40 50 60 70 80 70 60 50 40 30 20 10 0 50 80]  / 100*2^15)*2^-15"  TableDataTypeStr=fixdt(1,16,15)
  Rate Transition1 : RateTransition  Integrity=off  Deterministic=off
  Out1 : Outport
  wires:
  Rate Transition1/1 -> Buffer/1
  Counter Limited 0-1 @ 1.25Hz/1 -> Direct Lookup Table (n-D)/1
  Direct Lookup Table (n-D)/1 -> Rate Transition1/1
  Buffer/1 -> Out1/1

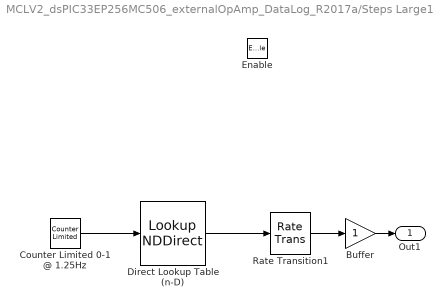
== system MCLV2_dsPIC33EP256MC506_externalOpAmp_DataLog_R2017a/Steps Large1 ==
  Enable : EnablePort  StatesWhenEnabling=reset
  Buffer : Gain  OutDataTypeStr=Inherit: Same as input  ParamDataTypeStr=Inherit: Same as input
  Counter Limited 0-1 @ 1.25Hz : simulink/Sources/Counter Limited  uplimit=19  tsamp=2.5
  Direct Lookup Table (n-D) : LookupNDDirect  NumberOfTableDimensions=1  Table="round([0 0 10 20 30 40 50 60 70 80 70 60 50 40 30 20 10 0 50 80]  / 100*2^15)*2^-15"  TableDataTypeStr=fixdt(1,16,15)
  Rate Transition1 : RateTransition  Integrity=off  Deterministic=off
  Out1 : Outport
  wires:
  Buffer/1 -> Out1/1
  Direct Lookup Table (n-D)/1 -> Rate Transition1/1
  Counter Limited 0-1 @ 1.25Hz/1 -> Direct Lookup Table (n-D)/1
  Rate Transition1/1 -> Buffer/1

== system MCLV2_dsPIC33EP256MC506_externalOpAmp_DataLog_R2017a/Timing Analysis ==
  note: Task 1 -> RB5 (PGD2)
      | Task 2 -> RB6 (PGC2)
      | Task 3 -> RF0 (HALL C)
      | Load: -> RC10  (HOME)
      | Overload -> LED 1
  MCU Load : MCHP_Blockset/Profiling/MCU Load  MCULoadPin=Dynamic Options  MCULoadPin_TXT=C10 / Pin[45]  MCULoadMeasure=off  TIMER_Resolution=Dynamic Options  TIMER_Resolution_TXT="Resol: 0.1143(us)  -  Max: 7.49(ms)"  MCHP_PORT={MCU Load Pin}{MCU_Load}0:1:C10;  MCHP_TIMER_REQUEST={MCU_Load}{MCU_Load}21:5:0:0:[]:524288;  MCHP_TIMER_RESULT=[1 65535 ]  MCHP_MASTERLINK=MCLV2_dsPIC33EP256MC506_externalOpAmp_DataLog_R2017a/Microchip Master  MCHP_COMPILED_INFO=CompiledSampleTime= [Inf Inf ];CompiledInportDataTypes=[ ];CompiledInportDataWidth=[];  Info="Timer 1:  Resol: 114.2857143(ns)  -  Max: 7.48983(ms)"  SampleTime=-1
      settings: SourceProductName=MPLAB Device Blocks for Simulink
  MCU Overload : MCHP_Blockset/Profiling/MCU Overload  MCUOverloadBlockOutput=off  MCUOverLoadPin=Dynamic Options  MCUOverLoadPin_TXT=D5 / Pin[53]  MCHP_PORT={OverLoad Pin}{OverLoad}0:1:D5;  MCHP_MASTERLINK=MCLV2_dsPIC33EP256MC506_externalOpAmp_DataLog_R2017a/Microchip Master  SampleTime=.1
      settings: SourceProductName=MPLAB Device Blocks for Simulink
  Tasks State : MCHP_Blockset/Profiling/Tasks State  TasksPin=[B5 B6 F0]  MCHP_PORT={Task D1 Running}{Task D1}15:1:B5;{Task D2 Running}{Task D2}15:1:B6;{Task D3 Running}{Task D3}15:1:F0;  MCHP_MASTERLINK=MCLV2_dsPIC33EP256MC506_externalOpAmp_DataLog_R2017a/Microchip Master
      settings: SourceProductName=MPLAB Device Blocks for Simulink

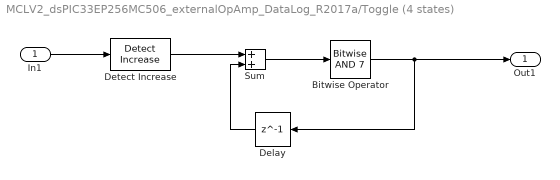
== system MCLV2_dsPIC33EP256MC506_externalOpAmp_DataLog_R2017a/Toggle (4 states) ==
  In1 : Inport
  Bitwise Operator : simulink/Logic and Bit Operations/Bitwise Operator  logicop=AND  UseBitMask=on  BitMask=7  BitMaskRealWorld=Stored Integer
  Delay : Delay  DelayLength=1  InitialCondition=0
  Detect Increase : simulink/Logic and Bit Operations/Detect Increase  vinit=1  OutDataTypeStr=boolean
  Sum : Sum  AccumDataTypeStr=uint16  OutDataTypeStr=uint16
  Out1 : Outport
  wires:
  Delay/1 -> Sum/2
  Sum/1 -> Bitwise Operator/1
  Detect Increase/1 -> Sum/1
  In1/1 -> Detect Increase/1
  Bitwise Operator/1 -> Out1/1, Delay/1

== system MCLV2_dsPIC33EP256MC506_externalOpAmp_DataLog_R2017a/MCLV2 with DC motor/Bias at rest ==
  In1 : Inport
  Enable : EnablePort
  LPF_3Hz : Subsystem  Tag=FilterWizardSubSystem
      settings: ErrorFcn=dspFilterRealizedInBasicElemsAlgLoopErrFcnCallback
  Out1 : Outport  InitialOutput=0
  wires:
  LPF_3Hz/1(Output) -> Out1/1
  In1/1 -> LPF_3Hz/1(Input)

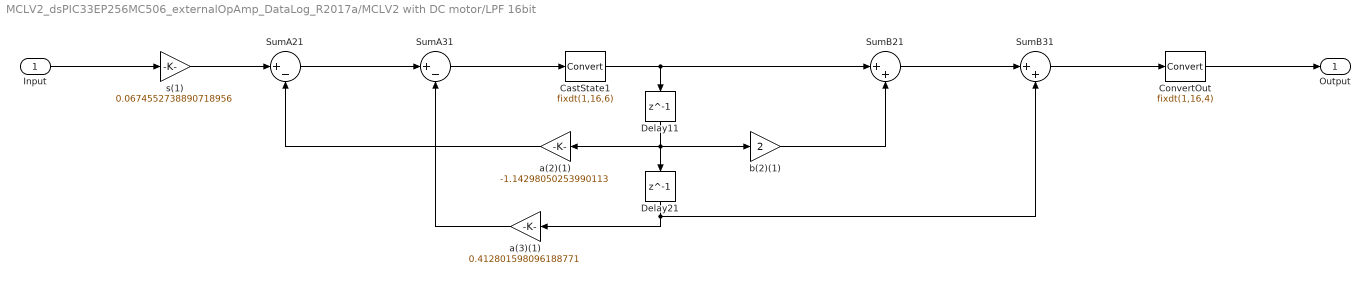
== system MCLV2_dsPIC33EP256MC506_externalOpAmp_DataLog_R2017a/MCLV2 with DC motor/LPF 16bit   ==
  Input : Inport
  CastState1 : DataTypeConversion  OutDataTypeStr=fixdt(1,16,6)
  ConvertOut : DataTypeConversion  OutDataTypeStr=fixdt(1,16,4)
  Delay11 : Delay  DelayLength=1  InitialCondition=0
  Delay21 : Delay  DelayLength=1  InitialCondition=0
  SumA21 : Sum  Inputs=|+-  AccumDataTypeStr=fixdt(1,16,6)  OutDataTypeStr=fixdt(1,16,6)
  SumA31 : Sum  Inputs=|+-  AccumDataTypeStr=fixdt(1,16,6)  OutDataTypeStr=fixdt(1,16,6)
  SumB21 : Sum  Inputs=|++  AccumDataTypeStr=fixdt(1,16,5)  OutDataTypeStr=fixdt(1,16,5)
  SumB31 : Sum  Inputs=|++  AccumDataTypeStr=fixdt(1,16,4)  OutDataTypeStr=fixdt(1,16,4)
  a(2)(1) : Gain  Gain=-1.14298050253990113  ParamDataTypeStr=fixdt(1,16,14)  OutDataTypeStr=fixdt(1,16,6)
  a(3)(1) : Gain  Gain=0.412801598096188771  ParamDataTypeStr=fixdt(0,16,17)  OutDataTypeStr=fixdt(1,16,8)
  b(2)(1) : Gain  Gain=2  ParamDataTypeStr=fixdt(0,16,14)  OutDataTypeStr=fixdt(1,16,5)
  s(1) : Gain  Gain=0.0674552738890718956  ParamDataTypeStr=fixdt(0,16,19)  OutDataTypeStr=fixdt(1,16,8)
  Output : Outport
  wires:
  Input/1 -> s(1)/1
  ConvertOut/1 -> Output/1
  Delay21/1 -> SumB31/2, a(3)(1)/1
  a(3)(1)/1 -> SumA31/2
  b(2)(1)/1 -> SumB21/2
  Delay11/1 -> Delay21/1, b(2)(1)/1, a(2)(1)/1
  a(2)(1)/1 -> SumA21/2
  SumB31/1 -> ConvertOut/1
  SumB21/1 -> SumB31/1
  CastState1/1 -> Delay11/1, SumB21/1
  SumA31/1 -> CastState1/1
  SumA21/1 -> SumA31/1
  s(1)/1 -> SumA21/1

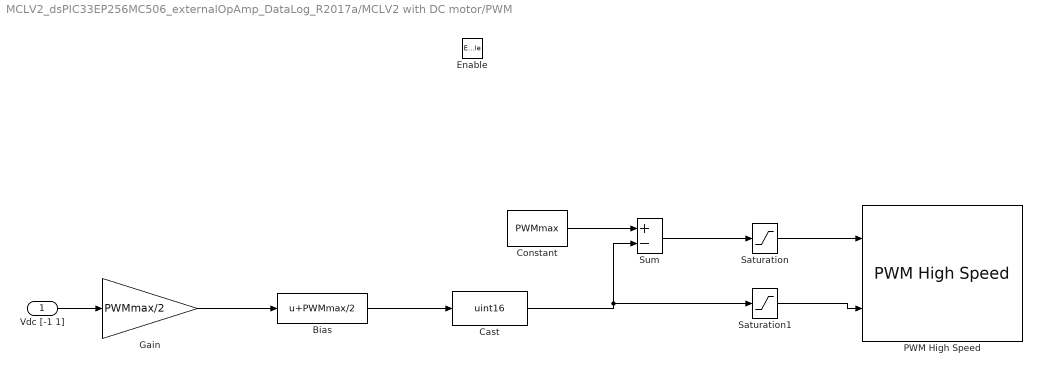
== system MCLV2_dsPIC33EP256MC506_externalOpAmp_DataLog_R2017a/MCLV2 with DC motor/PWM ==
  Vdc [-1 1] : Inport
  Enable : EnablePort
  Bias : Bias  Bias=PWMmax/2
  Cast : DataTypeConversion  OutDataTypeStr=uint16
  Constant : Constant  Value=PWMmax  OutDataTypeStr=uint16
  Gain : Gain  Gain=PWMmax/2  OutDataTypeStr=fixdt(1,32,1)
  PWM High Speed : MCHP_Blockset/PWM IO/PWM High Speed  pop1=[1]  chk1="[1  1  1  0  0]"  chkHL1="[1  1  0  1  1  1  1  1 ; 1  1  0  1  1  1  1  1]"  maxP1={ '50e-6','0.001','0.001','0.001','0.001','0.001','0.001','0.001';'0.001','0.001','1e-06','0.001','0.001','0.001','0.001','0.001'}  InitP2={ '50e-6','.001','0.001','0.001','0.001','0.001','0.001','0.001';'0.001','0.001','0.001','0.001','0.001','0.001','0.001','0.001'}  chkP2="[0  1  0  1  1  1  1  1 ; 1  0  0  1  1  1  1  1]"  InitDC={ '50','50','50','50','50','50','50','50';'0.001','0.001','0.001','50','50','50','50','50'}  chkDC="[1  1  1  1  1  1  1  1 ; 0  0  0  1  1  1  1  1]"  InitPh={ '0','0','0','0.001','0.001','0.001','0.001','0.001';'0','0','0','0.001','0.001','0.001','0.001','0.001'}  chkPh="[0  0  0  1  1  1  1  1 ; 0  0  0  1  1  1  1  1]"  edSEvTrigx={ '120e-9','-1','-1','-1','-1','-1','-1','-1'}  chkSEvTrigx="[0  1  1  1  1  1  1  1]"  popFlt="[2  2  1  1  1  1  1  1]"  popFltPin="[20  20  20   4   4   4   4   4]"  popFltPinRp="[1  1  1  1  1  1  1]"  popFltActivH="[2  2  1  1  1  1  1  1]"  popFltForceH="[2  2  2  2  2  2  2  2]"  popFltForceL="[1  1  1  1  1  1  1  1]"  chkFltBlkOut="[0  0  0  0  0  0  0  0]"  popIndepFaultMode="[1  1  1  1  1  1  1  1]"  popCurEnabled="[1  1  1  1  1  1  1  1]"  popCurPin="[4  31   4   4   4   4   4   4]"  popCurActiveH="[1  1  1  1  1  1  1  1]"  popCurForceH="[2  1  2  1  1  1  1  1]"  popCurForceL="[2  1  2  1  1  1  1  1]"  ChkCurBlkOut="[0  0  0  0  0  0  0  0]"  ChkCurBlkOutTime="[0  0  1  0  0  0  0  0]"  popBLANKSEL="[1  1  1  1  1  1  1  1]"  popBPHHBPHL="[1  1  1  1  1  1  1  1]"  popBPLHBPLL="[1  1  1  1  1  1  1  1]"  popFLTLEBEN_CLLEBEN="[1  1  1  1  1  1  1  1]"  popPHR_PHF="[2  1  1  1  1  1  1  1]"  popPLR_PLF="[3  1  1  1  1  1  1  1]"  edLEB={ '100e-9','50e-9','150e-9','50e-9','50e-9','50e-9','50e-9','50e-9'}  popDT="[1  1  1  3  3  3  3  3]"  edDTRx={ '0.02','1e-05','0.001','1e-05','1e-05','1e-05','1e-05','1e-05'}  edAltDTRx={ '0.5e-6','0.5e-6','0.5e-6','1e-05','1e-05','1e-05','1e-05','1e-05'}  S_INPUT="[5  5  5]"  S_INPUT_Size="[1  1  1]"  S_OUTPUT=[]  S_OUTPUT_Size=[]  S_DWORK_Type=[]  S_DWORK_Size=[]  ADC_VARTRIG={PWM Primary Special Event Trigger;6}  SampleTime=-1  ORDERING=None  MCHP_PORT={PWM1 Fault}{FLT32}4:0:B4;{PWM2 Fault}{FLT32}4:0:B4;{PWM1H}{PWM1H}4:4:B14;{PWM1L}{PWM1L}4:4:B15;{PWM2H}{PWM2H}4:4:B12;{PWM2L}{PWM2L}4:4:B13;  MCHP_MASTERLINK=MCLV2_dsPIC33EP256MC506_externalOpAmp_DataLog/Microchip Master  MCHP_VERSION=v3.39
      settings: SourceProductName=MPLAB Device Blocks for Simulink
  Saturation : Saturate  UpperLimit=PWMmax - (1e-6/50e-6)*PWMmax  LowerLimit=round( (0.5e-6/50e-6) *PWMmax )
  Saturation1 : Saturate  UpperLimit=PWMmax  LowerLimit=round( (0.5e-6/50e-6) *PWMmax )
  Sum : Sum  Inputs=+-  OutDataTypeStr=Inherit: Same as first input
  wires:
  Constant/1 -> Sum/1
  Vdc [-1 1]/1 -> Gain/1
  Saturation/1 -> PWM High Speed/1
  Bias/1 -> Cast/1
  Sum/1 -> Saturation/1
  Saturation1/1 -> PWM High Speed/2
  Cast/1 -> Saturation1/1, Sum/2
  Gain/1 -> Bias/1

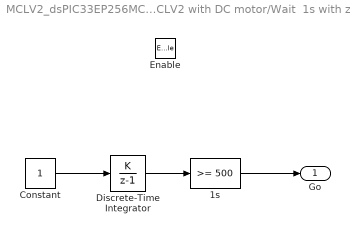
== system MCLV2_dsPIC33EP256MC506_externalOpAmp_DataLog_R2017a/MCLV2 with DC motor/Wait  1s with zero speed ==
  Enable : EnablePort
  "1s " : simulink/Logic and Bit Operations/Compare To Constant  relop=>=  const=500  OutDataTypeStr=boolean
  Constant : Constant  OutDataTypeStr=Inherit: Inherit via back propagation
  Discrete-Time Integrator : DiscreteIntegrator  IntegratorMethod=Accumulation: Forward Euler  gainval=1  InitialConditionSetting=State (most efficient)  SampleTime=-1  OutDataTypeStr=uint16  SaturateOnIntegerOverflow=on  ICPrevOutput=DiscIntNeverNeededParam  ICPrevScaledInput=DiscIntNeverNeededParam
  Go : Outport  InitialOutput=0
  wires:
  Discrete-Time Integrator/1 -> "1s "/1
  Constant/1 -> Discrete-Time Integrator/1
  "1s "/1 -> Go/1
